simulink model "c00010M_harness"  (R2018a)
settings: Solver=ode3  StartTime=0.0  StopTime=10.0  RelTol=1e-3  EnableMultiTasking=on
undefined symbols (not defined in the file): b, DiscIntNeverNeededParam, J, K, L, PosMinimaW3, R, sigbuilder_block
(part 18 of 43)

== system c00010M_harness/M036/Physical/W ==
  WIn : Inport
  DC_Engine : Subsystem
  Discrete-Time Integrator : DiscreteIntegrator  InitialCondition=5  SampleTime=-1  LimitOutput=on  UpperSaturationLimit=5  LowerSaturationLimit=0  ICPrevOutput=DiscIntNeverNeededParam  ICPrevScaledInput=DiscIntNeverNeededParam
  WPos : Outport
  wires:
  WIn/1 -> DC_Engine/1(input)
  DC_Engine/1(Speed) -> Discrete-Time Integrator/1
  Discrete-Time Integrator/1 -> WPos/1

== system c00010M_harness/M036/Physical/W5 ==
  WIn : Inport
  DC_Engine : Subsystem
  Discrete-Time Integrator : DiscreteIntegrator  InitialCondition=5  SampleTime=-1  LimitOutput=on  UpperSaturationLimit=5  LowerSaturationLimit=0  ICPrevOutput=DiscIntNeverNeededParam  ICPrevScaledInput=DiscIntNeverNeededParam
  WPos : Outport
  wires:
  Discrete-Time Integrator/1 -> WPos/1
  DC_Engine/1(Speed) -> Discrete-Time Integrator/1
  WIn/1 -> DC_Engine/1(input)

== system c00010M_harness/M036/Physical/W6 ==
  WIn : Inport
  DC_Engine : Subsystem
  Discrete-Time Integrator : DiscreteIntegrator  InitialCondition=5  SampleTime=-1  LimitOutput=on  UpperSaturationLimit=5  LowerSaturationLimit=PosMinimaW3  ICPrevOutput=DiscIntNeverNeededParam  ICPrevScaledInput=DiscIntNeverNeededParam
  WPos : Outport
  wires:
  WIn/1 -> DC_Engine/1(input)
  DC_Engine/1(Speed) -> Discrete-Time Integrator/1
  Discrete-Time Integrator/1 -> WPos/1

== system c00010M_harness/M037/Cyber/Pri ==
  D : Inport
  P : Inport  Port=2
  Switch : Switch  Criteria=u2 ~= 0
  User : Outport
  wires:
  Switch/1 -> User/1
  D/1 -> Switch/2, Switch/1
  P/1 -> Switch/3

== system c00010M_harness/M037/Cyber/Pri1 ==
  D : Inport
  P : Inport  Port=2
  P1 : Inport  Port=3
  Switch : Switch  Criteria=u2 ~= 0
  Switch1 : Switch  Criteria=u2 ~= 0
  User : Outport
  wires:
  Switch1/1 -> Switch/3
  D/1 -> Switch/2, Switch/1
  P/1 -> Switch1/2, Switch1/1
  Switch/1 -> User/1
  P1/1 -> Switch1/3

== system c00010M_harness/M037/Cyber/WL ==
  note: Sensors
  WPos : Inport
  User : Inport  Port=2
  OW : Inport  Port=3
  Chart : Stateflow chart  TreatAsAtomicUnit=on
  Constant : Constant  Value=-1
  Data Type Conversion : DataTypeConversion
  Switch : Switch  Criteria=u2 ~= 0  Threshold=1  ZeroCross=off
  WindowLogicOutput : Outport
  wires:
  Data Type Conversion/1 -> Switch/2
  Constant/1 -> Switch/1
  User/1 -> Chart/2(UI)
  WPos/1 -> Chart/1(S)
  Switch/1 -> WindowLogicOutput/1
  OW/1 -> Data Type Conversion/1
  Chart/1(W) -> Switch/3

== system c00010M_harness/M037/Cyber/WL1 ==
  note: Sensors
  WPos : Inport
  User : Inport  Port=2
  OW : Inport  Port=3
  Chart1 : Stateflow chart  TreatAsAtomicUnit=on
  Constant : Constant  Value=-1
  Data Type Conversion : DataTypeConversion
  Switch : Switch  Criteria=u2 ~= 0  Threshold=1  ZeroCross=off
  WindowLogicOutput : Outport
  wires:
  OW/1 -> Data Type Conversion/1
  Switch/1 -> WindowLogicOutput/1
  WPos/1 -> Chart1/1(S)
  User/1 -> Chart1/2(UI)
  Constant/1 -> Switch/1
  Data Type Conversion/1 -> Switch/2
  Chart1/1(W) -> Switch/3

== system c00010M_harness/M037/Cyber/WL2 ==
  note: Sensors
  WPos : Inport
  User : Inport  Port=2
  OW : Inport  Port=3
  L : Inport  Port=4
  Chart1 : Stateflow chart  TreatAsAtomicUnit=on
  Constant : Constant  Value=-1
  Constant1 : Constant  Value=0
  Constant2 : Constant  Value=PosMinimaW3
  Data Type Conversion : DataTypeConversion
  Switch : Switch  Criteria=u2 ~= 0  Threshold=1  ZeroCross=off
  Switch1 : Switch  Criteria=u2 ~= 0
  WindowLogicOutput : Outport
  wires:
  Constant2/1 -> Chart1/3(PosMinW3)
  L/1 -> Switch1/2
  Data Type Conversion/1 -> Switch/2
  Constant/1 -> Switch/1
  Chart1/1(W) -> Switch1/3
  User/1 -> Chart1/2(UI)
  WPos/1 -> Chart1/1(S)
  Switch1/1 -> Switch/3
  Constant1/1 -> Switch1/1
  Switch/1 -> WindowLogicOutput/1
  OW/1 -> Data Type Conversion/1

== system c00010M_harness/M037/Physical/W ==
  WIn : Inport
  DC_Engine : Subsystem
  Discrete-Time Integrator : DiscreteIntegrator  InitialCondition=5  SampleTime=-1  LimitOutput=on  UpperSaturationLimit=5  LowerSaturationLimit=0  ICPrevOutput=DiscIntNeverNeededParam  ICPrevScaledInput=DiscIntNeverNeededParam
  WPos : Outport
  wires:
  WIn/1 -> DC_Engine/1(input)
  DC_Engine/1(Speed) -> Discrete-Time Integrator/1
  Discrete-Time Integrator/1 -> WPos/1

== system c00010M_harness/M037/Physical/W5 ==
  WIn : Inport
  DC_Engine : Subsystem
  Discrete-Time Integrator : DiscreteIntegrator  InitialCondition=5  SampleTime=-1  LimitOutput=on  UpperSaturationLimit=5  LowerSaturationLimit=0  ICPrevOutput=DiscIntNeverNeededParam  ICPrevScaledInput=DiscIntNeverNeededParam
  WPos : Outport
  wires:
  Discrete-Time Integrator/1 -> WPos/1
  DC_Engine/1(Speed) -> Discrete-Time Integrator/1
  WIn/1 -> DC_Engine/1(input)

== system c00010M_harness/M037/Physical/W6 ==
  WIn : Inport
  DC_Engine : Subsystem
  Discrete-Time Integrator : DiscreteIntegrator  InitialCondition=5  SampleTime=-1  LimitOutput=on  UpperSaturationLimit=5  LowerSaturationLimit=PosMinimaW3  ICPrevOutput=DiscIntNeverNeededParam  ICPrevScaledInput=DiscIntNeverNeededParam
  WPos : Outport
  wires:
  WIn/1 -> DC_Engine/1(input)
  DC_Engine/1(Speed) -> Discrete-Time Integrator/1
  Discrete-Time Integrator/1 -> WPos/1

== system c00010M_harness/M039/Cyber/Pri ==
  D : Inport
  P : Inport  Port=2
  Switch : Switch  Criteria=u2 ~= 0
  User : Outport
  wires:
  Switch/1 -> User/1
  D/1 -> Switch/2, Switch/1
  P/1 -> Switch/3

== system c00010M_harness/M039/Cyber/Pri1 ==
  D : Inport
  P : Inport  Port=2
  P1 : Inport  Port=3
  Switch : Switch  Criteria=u2 ~= 0
  Switch1 : Switch  Criteria=u2 ~= 0
  User : Outport
  wires:
  Switch1/1 -> Switch/3
  D/1 -> Switch/2, Switch/1
  P/1 -> Switch1/2, Switch1/1
  Switch/1 -> User/1
  P1/1 -> Switch1/3

== system c00010M_harness/M039/Cyber/WL ==
  note: Sensors
  WPos : Inport
  User : Inport  Port=2
  OW : Inport  Port=3
  Chart : Stateflow chart  TreatAsAtomicUnit=on
  Constant : Constant  Value=-1
  Data Type Conversion : DataTypeConversion
  Switch : Switch  Criteria=u2 ~= 0  Threshold=1  ZeroCross=off
  WindowLogicOutput : Outport
  wires:
  Data Type Conversion/1 -> Switch/2
  Constant/1 -> Switch/1
  User/1 -> Chart/2(UI)
  WPos/1 -> Chart/1(S)
  Switch/1 -> WindowLogicOutput/1
  OW/1 -> Data Type Conversion/1
  Chart/1(W) -> Switch/3

== system c00010M_harness/M039/Cyber/WL1 ==
  note: Sensors
  WPos : Inport
  User : Inport  Port=2
  OW : Inport  Port=3
  Chart1 : Stateflow chart  TreatAsAtomicUnit=on
  Constant : Constant  Value=-1
  Data Type Conversion : DataTypeConversion
  Switch : Switch  Criteria=u2 ~= 0  Threshold=1  ZeroCross=off
  WindowLogicOutput : Outport
  wires:
  OW/1 -> Data Type Conversion/1
  Switch/1 -> WindowLogicOutput/1
  WPos/1 -> Chart1/1(S)
  User/1 -> Chart1/2(UI)
  Constant/1 -> Switch/1
  Data Type Conversion/1 -> Switch/2
  Chart1/1(W) -> Switch/3

== system c00010M_harness/M039/Cyber/WL2 ==
  note: Sensors
  WPos : Inport
  User : Inport  Port=2
  OW : Inport  Port=3
  L : Inport  Port=4
  Chart1 : Stateflow chart  TreatAsAtomicUnit=on
  Constant : Constant  Value=-1
  Constant1 : Constant  Value=0
  Constant2 : Constant  Value=PosMinimaW3
  Data Type Conversion : DataTypeConversion
  Switch : Switch  Criteria=u2 ~= 0  Threshold=1  ZeroCross=off
  Switch1 : Switch  Criteria=u2 ~= 0
  WindowLogicOutput : Outport
  wires:
  Constant2/1 -> Chart1/3(PosMinW3)
  L/1 -> Switch1/2
  Data Type Conversion/1 -> Switch/2
  Constant/1 -> Switch/1
  Chart1/1(W) -> Switch1/3
  User/1 -> Chart1/2(UI)
  WPos/1 -> Chart1/1(S)
  Switch1/1 -> Switch/3
  Constant1/1 -> Switch1/1
  Switch/1 -> WindowLogicOutput/1
  OW/1 -> Data Type Conversion/1

== system c00010M_harness/M039/Physical/W ==
  WIn : Inport
  DC_Engine : Subsystem
  Discrete-Time Integrator : DiscreteIntegrator  InitialCondition=5  SampleTime=-1  LimitOutput=on  UpperSaturationLimit=5  LowerSaturationLimit=0  ICPrevOutput=DiscIntNeverNeededParam  ICPrevScaledInput=DiscIntNeverNeededParam
  WPos : Outport
  wires:
  WIn/1 -> DC_Engine/1(input)
  DC_Engine/1(Speed) -> Discrete-Time Integrator/1
  Discrete-Time Integrator/1 -> WPos/1

== system c00010M_harness/M039/Physical/W5 ==
  WIn : Inport
  DC_Engine : Subsystem
  Discrete-Time Integrator : DiscreteIntegrator  InitialCondition=5  SampleTime=-1  LimitOutput=on  UpperSaturationLimit=5  LowerSaturationLimit=0  ICPrevOutput=DiscIntNeverNeededParam  ICPrevScaledInput=DiscIntNeverNeededParam
  WPos : Outport
  wires:
  Discrete-Time Integrator/1 -> WPos/1
  DC_Engine/1(Speed) -> Discrete-Time Integrator/1
  WIn/1 -> DC_Engine/1(input)

== system c00010M_harness/M039/Physical/W6 ==
  WIn : Inport
  DC_Engine : Subsystem
  Discrete-Time Integrator : DiscreteIntegrator  InitialCondition=5  SampleTime=-1  LimitOutput=on  UpperSaturationLimit=5  LowerSaturationLimit=PosMinimaW3  ICPrevOutput=DiscIntNeverNeededParam  ICPrevScaledInput=DiscIntNeverNeededParam
  WPos : Outport
  wires:
  WIn/1 -> DC_Engine/1(input)
  DC_Engine/1(Speed) -> Discrete-Time Integrator/1
  Discrete-Time Integrator/1 -> WPos/1

== system c00010M_harness/M040/Cyber/Pri ==
  D : Inport
  P : Inport  Port=2
  Switch : Switch  Criteria=u2 ~= 0
  User : Outport
  wires:
  Switch/1 -> User/1
  D/1 -> Switch/2, Switch/1
  P/1 -> Switch/3

== system c00010M_harness/M040/Cyber/Pri1 ==
  D : Inport
  P : Inport  Port=2
  P1 : Inport  Port=3
  Switch : Switch  Criteria=u2 ~= 0
  Switch1 : Switch  Criteria=u2 ~= 0
  User : Outport
  wires:
  Switch1/1 -> Switch/3
  D/1 -> Switch/2, Switch/1
  P/1 -> Switch1/2, Switch1/1
  Switch/1 -> User/1
  P1/1 -> Switch1/3

== system c00010M_harness/M040/Cyber/WL ==
  note: Sensors
  WPos : Inport
  User : Inport  Port=2
  OW : Inport  Port=3
  Chart : Stateflow chart  TreatAsAtomicUnit=on
  Constant : Constant  Value=-1
  Data Type Conversion : DataTypeConversion
  Switch : Switch  Criteria=u2 ~= 0  Threshold=1  ZeroCross=off
  WindowLogicOutput : Outport
  wires:
  Data Type Conversion/1 -> Switch/2
  Constant/1 -> Switch/1
  User/1 -> Chart/2(UI)
  WPos/1 -> Chart/1(S)
  Switch/1 -> WindowLogicOutput/1
  OW/1 -> Data Type Conversion/1
  Chart/1(W) -> Switch/3

== system c00010M_harness/M040/Cyber/WL1 ==
  note: Sensors
  WPos : Inport
  User : Inport  Port=2
  OW : Inport  Port=3
  Chart1 : Stateflow chart  TreatAsAtomicUnit=on
  Constant : Constant  Value=-1
  Data Type Conversion : DataTypeConversion
  Switch : Switch  Criteria=u2 ~= 0  Threshold=1  ZeroCross=off
  WindowLogicOutput : Outport
  wires:
  OW/1 -> Data Type Conversion/1
  Switch/1 -> WindowLogicOutput/1
  WPos/1 -> Chart1/1(S)
  User/1 -> Chart1/2(UI)
  Constant/1 -> Switch/1
  Data Type Conversion/1 -> Switch/2
  Chart1/1(W) -> Switch/3

== system c00010M_harness/M040/Cyber/WL2 ==
  note: Sensors
  WPos : Inport
  User : Inport  Port=2
  OW : Inport  Port=3
  L : Inport  Port=4
  Chart1 : Stateflow chart  TreatAsAtomicUnit=on
  Constant : Constant  Value=-1
  Constant1 : Constant  Value=0
  Constant2 : Constant  Value=PosMinimaW3
  Data Type Conversion : DataTypeConversion
  Switch : Switch  Criteria=u2 ~= 0  Threshold=1  ZeroCross=off
  Switch1 : Switch  Criteria=u2 ~= 0
  WindowLogicOutput : Outport
  wires:
  Constant2/1 -> Chart1/3(PosMinW3)
  L/1 -> Switch1/2
  Data Type Conversion/1 -> Switch/2
  Constant/1 -> Switch/1
  Chart1/1(W) -> Switch1/3
  User/1 -> Chart1/2(UI)
  WPos/1 -> Chart1/1(S)
  Switch1/1 -> Switch/3
  Constant1/1 -> Switch1/1
  Switch/1 -> WindowLogicOutput/1
  OW/1 -> Data Type Conversion/1

== system c00010M_harness/M040/Physical/W ==
  WIn : Inport
  DC_Engine : Subsystem
  Discrete-Time Integrator : DiscreteIntegrator  InitialCondition=5  SampleTime=-1  LimitOutput=on  UpperSaturationLimit=5  LowerSaturationLimit=0  ICPrevOutput=DiscIntNeverNeededParam  ICPrevScaledInput=DiscIntNeverNeededParam
  WPos : Outport
  wires:
  WIn/1 -> DC_Engine/1(input)
  DC_Engine/1(Speed) -> Discrete-Time Integrator/1
  Discrete-Time Integrator/1 -> WPos/1

== system c00010M_harness/M040/Physical/W5 ==
  WIn : Inport
  DC_Engine : Subsystem
  Discrete-Time Integrator : DiscreteIntegrator  InitialCondition=5  SampleTime=-1  LimitOutput=on  UpperSaturationLimit=5  LowerSaturationLimit=0  ICPrevOutput=DiscIntNeverNeededParam  ICPrevScaledInput=DiscIntNeverNeededParam
  WPos : Outport
  wires:
  Discrete-Time Integrator/1 -> WPos/1
  DC_Engine/1(Speed) -> Discrete-Time Integrator/1
  WIn/1 -> DC_Engine/1(input)

== system c00010M_harness/M040/Physical/W6 ==
  WIn : Inport
  DC_Engine : Subsystem
  Discrete-Time Integrator : DiscreteIntegrator  InitialCondition=5  SampleTime=-1  LimitOutput=on  UpperSaturationLimit=5  LowerSaturationLimit=PosMinimaW3  ICPrevOutput=DiscIntNeverNeededParam  ICPrevScaledInput=DiscIntNeverNeededParam
  WPos : Outport
  wires:
  WIn/1 -> DC_Engine/1(input)
  DC_Engine/1(Speed) -> Discrete-Time Integrator/1
  Discrete-Time Integrator/1 -> WPos/1

== system c00010M_harness/M041/Cyber/Pri ==
  D : Inport
  P : Inport  Port=2
  Switch : Switch  Criteria=u2 ~= 0
  User : Outport
  wires:
  Switch/1 -> User/1
  D/1 -> Switch/2, Switch/1
  P/1 -> Switch/3

== system c00010M_harness/M041/Cyber/Pri1 ==
  D : Inport
  P : Inport  Port=2
  P1 : Inport  Port=3
  Switch : Switch  Criteria=u2 ~= 0
  Switch1 : Switch  Criteria=u2 ~= 0
  User : Outport
  wires:
  Switch1/1 -> Switch/3
  D/1 -> Switch/2, Switch/1
  P/1 -> Switch1/2, Switch1/1
  Switch/1 -> User/1
  P1/1 -> Switch1/3

== system c00010M_harness/M041/Cyber/WL ==
  note: Sensors
  WPos : Inport
  User : Inport  Port=2
  OW : Inport  Port=3
  Chart : Stateflow chart  TreatAsAtomicUnit=on
  Constant : Constant  Value=-1
  Data Type Conversion : DataTypeConversion
  Switch : Switch  Criteria=u2 ~= 0  Threshold=1  ZeroCross=off
  WindowLogicOutput : Outport
  wires:
  Data Type Conversion/1 -> Switch/2
  Constant/1 -> Switch/1
  User/1 -> Chart/2(UI)
  WPos/1 -> Chart/1(S)
  Switch/1 -> WindowLogicOutput/1
  OW/1 -> Data Type Conversion/1
  Chart/1(W) -> Switch/3

== system c00010M_harness/M041/Cyber/WL1 ==
  note: Sensors
  WPos : Inport
  User : Inport  Port=2
  OW : Inport  Port=3
  Chart1 : Stateflow chart  TreatAsAtomicUnit=on
  Constant : Constant  Value=-1
  Data Type Conversion : DataTypeConversion
  Switch : Switch  Criteria=u2 ~= 0  Threshold=1  ZeroCross=off
  WindowLogicOutput : Outport
  wires:
  OW/1 -> Data Type Conversion/1
  Switch/1 -> WindowLogicOutput/1
  WPos/1 -> Chart1/1(S)
  User/1 -> Chart1/2(UI)
  Constant/1 -> Switch/1
  Data Type Conversion/1 -> Switch/2
  Chart1/1(W) -> Switch/3

== system c00010M_harness/M041/Cyber/WL2 ==
  note: Sensors
  WPos : Inport
  User : Inport  Port=2
  OW : Inport  Port=3
  L : Inport  Port=4
  Chart1 : Stateflow chart  TreatAsAtomicUnit=on
  Constant : Constant  Value=-1
  Constant1 : Constant  Value=0
  Constant2 : Constant  Value=PosMinimaW3
  Data Type Conversion : DataTypeConversion
  Switch : Switch  Criteria=u2 ~= 0  Threshold=1  ZeroCross=off
  Switch1 : Switch  Criteria=u2 ~= 0
  WindowLogicOutput : Outport
  wires:
  Constant2/1 -> Chart1/3(PosMinW3)
  L/1 -> Switch1/2
  Data Type Conversion/1 -> Switch/2
  Constant/1 -> Switch/1
  Chart1/1(W) -> Switch1/3
  User/1 -> Chart1/2(UI)
  WPos/1 -> Chart1/1(S)
  Switch1/1 -> Switch/3
  Constant1/1 -> Switch1/1
  Switch/1 -> WindowLogicOutput/1
  OW/1 -> Data Type Conversion/1

== system c00010M_harness/M041/Physical/W ==
  WIn : Inport
  DC_Engine : Subsystem
  Discrete-Time Integrator : DiscreteIntegrator  InitialCondition=5  SampleTime=-1  LimitOutput=on  UpperSaturationLimit=5  LowerSaturationLimit=0  ICPrevOutput=DiscIntNeverNeededParam  ICPrevScaledInput=DiscIntNeverNeededParam
  WPos : Outport
  wires:
  WIn/1 -> DC_Engine/1(input)
  DC_Engine/1(Speed) -> Discrete-Time Integrator/1
  Discrete-Time Integrator/1 -> WPos/1

== system c00010M_harness/M041/Physical/W5 ==
  WIn : Inport
  DC_Engine : Subsystem
  Discrete-Time Integrator : DiscreteIntegrator  InitialCondition=5  SampleTime=-1  LimitOutput=on  UpperSaturationLimit=5  LowerSaturationLimit=0  ICPrevOutput=DiscIntNeverNeededParam  ICPrevScaledInput=DiscIntNeverNeededParam
  WPos : Outport
  wires:
  Discrete-Time Integrator/1 -> WPos/1
  DC_Engine/1(Speed) -> Discrete-Time Integrator/1
  WIn/1 -> DC_Engine/1(input)

== system c00010M_harness/M041/Physical/W6 ==
  WIn : Inport
  DC_Engine : Subsystem
  Discrete-Time Integrator : DiscreteIntegrator  InitialCondition=5  SampleTime=-1  LimitOutput=on  UpperSaturationLimit=5  LowerSaturationLimit=PosMinimaW3  ICPrevOutput=DiscIntNeverNeededParam  ICPrevScaledInput=DiscIntNeverNeededParam
  WPos : Outport
  wires:
  WIn/1 -> DC_Engine/1(input)
  DC_Engine/1(Speed) -> Discrete-Time Integrator/1
  Discrete-Time Integrator/1 -> WPos/1

== system c00010M_harness/M043/Cyber/Pri ==
  D : Inport
  P : Inport  Port=2
  Switch : Switch  Criteria=u2 ~= 0
  User : Outport
  wires:
  Switch/1 -> User/1
  D/1 -> Switch/2, Switch/1
  P/1 -> Switch/3

== system c00010M_harness/M043/Cyber/Pri1 ==
  D : Inport
  P : Inport  Port=2
  P1 : Inport  Port=3
  Switch : Switch  Criteria=u2 ~= 0
  Switch1 : Switch  Criteria=u2 ~= 0
  User : Outport
  wires:
  Switch1/1 -> Switch/3
  D/1 -> Switch/2, Switch/1
  P/1 -> Switch1/2, Switch1/1
  Switch/1 -> User/1
  P1/1 -> Switch1/3

== system c00010M_harness/M043/Cyber/WL ==
  note: Sensors
  WPos : Inport
  User : Inport  Port=2
  OW : Inport  Port=3
  Chart : Stateflow chart  TreatAsAtomicUnit=on
  Constant : Constant  Value=-1
  Data Type Conversion : DataTypeConversion
  Switch : Switch  Criteria=u2 ~= 0  Threshold=1  ZeroCross=off
  WindowLogicOutput : Outport
  wires:
  Data Type Conversion/1 -> Switch/2
  Constant/1 -> Switch/1
  User/1 -> Chart/2(UI)
  WPos/1 -> Chart/1(S)
  Switch/1 -> WindowLogicOutput/1
  OW/1 -> Data Type Conversion/1
  Chart/1(W) -> Switch/3

== system c00010M_harness/M043/Cyber/WL1 ==
  note: Sensors
  WPos : Inport
  User : Inport  Port=2
  OW : Inport  Port=3
  Chart1 : Stateflow chart  TreatAsAtomicUnit=on
  Constant : Constant  Value=-1
  Data Type Conversion : DataTypeConversion
  Switch : Switch  Criteria=u2 ~= 0  Threshold=1  ZeroCross=off
  WindowLogicOutput : Outport
  wires:
  OW/1 -> Data Type Conversion/1
  Switch/1 -> WindowLogicOutput/1
  WPos/1 -> Chart1/1(S)
  User/1 -> Chart1/2(UI)
  Constant/1 -> Switch/1
  Data Type Conversion/1 -> Switch/2
  Chart1/1(W) -> Switch/3

== system c00010M_harness/M043/Cyber/WL2 ==
  note: Sensors
  WPos : Inport
  User : Inport  Port=2
  OW : Inport  Port=3
  L : Inport  Port=4
  Chart1 : Stateflow chart  TreatAsAtomicUnit=on
  Constant : Constant  Value=-1
  Constant1 : Constant  Value=0
  Constant2 : Constant  Value=PosMinimaW3
  Data Type Conversion : DataTypeConversion
  Switch : Switch  Criteria=u2 ~= 0  Threshold=1  ZeroCross=off
  Switch1 : Switch  Criteria=u2 ~= 0
  WindowLogicOutput : Outport
  wires:
  Constant2/1 -> Chart1/3(PosMinW3)
  L/1 -> Switch1/2
  Data Type Conversion/1 -> Switch/2
  Constant/1 -> Switch/1
  Chart1/1(W) -> Switch1/3
  User/1 -> Chart1/2(UI)
  WPos/1 -> Chart1/1(S)
  Switch1/1 -> Switch/3
  Constant1/1 -> Switch1/1
  Switch/1 -> WindowLogicOutput/1
  OW/1 -> Data Type Conversion/1

== system c00010M_harness/M043/Physical/W ==
  WIn : Inport
  DC_Engine : Subsystem
  Discrete-Time Integrator : DiscreteIntegrator  InitialCondition=5  SampleTime=-1  LimitOutput=on  UpperSaturationLimit=5  LowerSaturationLimit=0  ICPrevOutput=DiscIntNeverNeededParam  ICPrevScaledInput=DiscIntNeverNeededParam
  WPos : Outport
  wires:
  WIn/1 -> DC_Engine/1(input)
  DC_Engine/1(Speed) -> Discrete-Time Integrator/1
  Discrete-Time Integrator/1 -> WPos/1

== system c00010M_harness/M043/Physical/W5 ==
  WIn : Inport
  DC_Engine : Subsystem
  Discrete-Time Integrator : DiscreteIntegrator  InitialCondition=5  SampleTime=-1  LimitOutput=on  UpperSaturationLimit=5  LowerSaturationLimit=0  ICPrevOutput=DiscIntNeverNeededParam  ICPrevScaledInput=DiscIntNeverNeededParam
  WPos : Outport
  wires:
  Discrete-Time Integrator/1 -> WPos/1
  DC_Engine/1(Speed) -> Discrete-Time Integrator/1
  WIn/1 -> DC_Engine/1(input)

== system c00010M_harness/M043/Physical/W6 ==
  WIn : Inport
  DC_Engine : Subsystem
  Discrete-Time Integrator : DiscreteIntegrator  InitialCondition=5  SampleTime=-1  LimitOutput=on  UpperSaturationLimit=5  LowerSaturationLimit=PosMinimaW3  ICPrevOutput=DiscIntNeverNeededParam  ICPrevScaledInput=DiscIntNeverNeededParam
  WPos : Outport
  wires:
  WIn/1 -> DC_Engine/1(input)
  DC_Engine/1(Speed) -> Discrete-Time Integrator/1
  Discrete-Time Integrator/1 -> WPos/1

== system c00010M_harness/M044/Cyber/Pri ==
  D : Inport
  P : Inport  Port=2
  Switch : Switch  Criteria=u2 ~= 0
  User : Outport
  wires:
  Switch/1 -> User/1
  D/1 -> Switch/2, Switch/1
  P/1 -> Switch/3

== system c00010M_harness/M044/Cyber/Pri1 ==
  D : Inport
  P : Inport  Port=2
  P1 : Inport  Port=3
  Switch : Switch  Criteria=u2 ~= 0
  Switch1 : Switch  Criteria=u2 ~= 0
  User : Outport
  wires:
  Switch1/1 -> Switch/3
  D/1 -> Switch/2, Switch/1
  P/1 -> Switch1/2, Switch1/1
  Switch/1 -> User/1
  P1/1 -> Switch1/3

== system c00010M_harness/M044/Cyber/WL ==
  note: Sensors
  WPos : Inport
  User : Inport  Port=2
  OW : Inport  Port=3
  Chart : Stateflow chart  TreatAsAtomicUnit=on
  Constant : Constant  Value=-1
  Data Type Conversion : DataTypeConversion
  Switch : Switch  Criteria=u2 ~= 0  Threshold=1  ZeroCross=off
  WindowLogicOutput : Outport
  wires:
  Data Type Conversion/1 -> Switch/2
  Constant/1 -> Switch/1
  User/1 -> Chart/2(UI)
  WPos/1 -> Chart/1(S)
  Switch/1 -> WindowLogicOutput/1
  OW/1 -> Data Type Conversion/1
  Chart/1(W) -> Switch/3

== system c00010M_harness/M044/Cyber/WL1 ==
  note: Sensors
  WPos : Inport
  User : Inport  Port=2
  OW : Inport  Port=3
  Chart1 : Stateflow chart  TreatAsAtomicUnit=on
  Constant : Constant  Value=-1
  Data Type Conversion : DataTypeConversion
  Switch : Switch  Criteria=u2 ~= 0  Threshold=1  ZeroCross=off
  WindowLogicOutput : Outport
  wires:
  OW/1 -> Data Type Conversion/1
  Switch/1 -> WindowLogicOutput/1
  WPos/1 -> Chart1/1(S)
  User/1 -> Chart1/2(UI)
  Constant/1 -> Switch/1
  Data Type Conversion/1 -> Switch/2
  Chart1/1(W) -> Switch/3

== system c00010M_harness/M044/Cyber/WL2 ==
  note: Sensors
  WPos : Inport
  User : Inport  Port=2
  OW : Inport  Port=3
  L : Inport  Port=4
  Chart1 : Stateflow chart  TreatAsAtomicUnit=on
  Constant : Constant  Value=-1
  Constant1 : Constant  Value=0
  Constant2 : Constant  Value=PosMinimaW3
  Data Type Conversion : DataTypeConversion
  Switch : Switch  Criteria=u2 ~= 0  Threshold=1  ZeroCross=off
  Switch1 : Switch  Criteria=u2 ~= 0
  WindowLogicOutput : Outport
  wires:
  Constant2/1 -> Chart1/3(PosMinW3)
  L/1 -> Switch1/2
  Data Type Conversion/1 -> Switch/2
  Constant/1 -> Switch/1
  Chart1/1(W) -> Switch1/3
  User/1 -> Chart1/2(UI)
  WPos/1 -> Chart1/1(S)
  Switch1/1 -> Switch/3
  Constant1/1 -> Switch1/1
  Switch/1 -> WindowLogicOutput/1
  OW/1 -> Data Type Conversion/1

== system c00010M_harness/M044/Physical/W ==
  WIn : Inport
  DC_Engine : Subsystem
  Discrete-Time Integrator : DiscreteIntegrator  InitialCondition=5  SampleTime=-1  LimitOutput=on  UpperSaturationLimit=5  LowerSaturationLimit=0  ICPrevOutput=DiscIntNeverNeededParam  ICPrevScaledInput=DiscIntNeverNeededParam
  WPos : Outport
  wires:
  WIn/1 -> DC_Engine/1(input)
  DC_Engine/1(Speed) -> Discrete-Time Integrator/1
  Discrete-Time Integrator/1 -> WPos/1

== system c00010M_harness/M044/Physical/W5 ==
  WIn : Inport
  DC_Engine : Subsystem
  Discrete-Time Integrator : DiscreteIntegrator  InitialCondition=5  SampleTime=-1  LimitOutput=on  UpperSaturationLimit=5  LowerSaturationLimit=0  ICPrevOutput=DiscIntNeverNeededParam  ICPrevScaledInput=DiscIntNeverNeededParam
  WPos : Outport
  wires:
  Discrete-Time Integrator/1 -> WPos/1
  DC_Engine/1(Speed) -> Discrete-Time Integrator/1
  WIn/1 -> DC_Engine/1(input)

== system c00010M_harness/M044/Physical/W6 ==
  WIn : Inport
  DC_Engine : Subsystem
  Discrete-Time Integrator : DiscreteIntegrator  InitialCondition=5  SampleTime=-1  LimitOutput=on  UpperSaturationLimit=5  LowerSaturationLimit=PosMinimaW3  ICPrevOutput=DiscIntNeverNeededParam  ICPrevScaledInput=DiscIntNeverNeededParam
  WPos : Outport
  wires:
  WIn/1 -> DC_Engine/1(input)
  DC_Engine/1(Speed) -> Discrete-Time Integrator/1
  Discrete-Time Integrator/1 -> WPos/1

== system c00010M_harness/M045/Cyber/Pri ==
  D : Inport
  P : Inport  Port=2
  Switch : Switch  Criteria=u2 ~= 0
  User : Outport
  wires:
  Switch/1 -> User/1
  D/1 -> Switch/2, Switch/1
  P/1 -> Switch/3

== system c00010M_harness/M045/Cyber/Pri1 ==
  D : Inport
  P : Inport  Port=2
  P1 : Inport  Port=3
  Switch : Switch  Criteria=u2 ~= 0
  Switch1 : Switch  Criteria=u2 ~= 0
  User : Outport
  wires:
  Switch1/1 -> Switch/3
  D/1 -> Switch/2, Switch/1
  P/1 -> Switch1/2, Switch1/1
  Switch/1 -> User/1
  P1/1 -> Switch1/3

== system c00010M_harness/M045/Cyber/WL ==
  note: Sensors
  WPos : Inport
  User : Inport  Port=2
  OW : Inport  Port=3
  Chart : Stateflow chart  TreatAsAtomicUnit=on
  Constant : Constant  Value=-1
  Data Type Conversion : DataTypeConversion
  Switch : Switch  Criteria=u2 ~= 0  Threshold=1  ZeroCross=off
  WindowLogicOutput : Outport
  wires:
  Data Type Conversion/1 -> Switch/2
  Constant/1 -> Switch/1
  User/1 -> Chart/2(UI)
  WPos/1 -> Chart/1(S)
  Switch/1 -> WindowLogicOutput/1
  OW/1 -> Data Type Conversion/1
  Chart/1(W) -> Switch/3

== system c00010M_harness/M045/Cyber/WL1 ==
  note: Sensors
  WPos : Inport
  User : Inport  Port=2
  OW : Inport  Port=3
  Chart1 : Stateflow chart  TreatAsAtomicUnit=on
  Constant : Constant  Value=-1
  Data Type Conversion : DataTypeConversion
  Switch : Switch  Criteria=u2 ~= 0  Threshold=1  ZeroCross=off
  WindowLogicOutput : Outport
  wires:
  OW/1 -> Data Type Conversion/1
  Switch/1 -> WindowLogicOutput/1
  WPos/1 -> Chart1/1(S)
  User/1 -> Chart1/2(UI)
  Constant/1 -> Switch/1
  Data Type Conversion/1 -> Switch/2
  Chart1/1(W) -> Switch/3

== system c00010M_harness/M045/Cyber/WL2 ==
  note: Sensors
  WPos : Inport
  User : Inport  Port=2
  OW : Inport  Port=3
  L : Inport  Port=4
  Chart1 : Stateflow chart  TreatAsAtomicUnit=on
  Constant : Constant  Value=-1
  Constant1 : Constant  Value=0
  Constant2 : Constant  Value=PosMinimaW3
  Data Type Conversion : DataTypeConversion
  Switch : Switch  Criteria=u2 ~= 0  Threshold=1  ZeroCross=off
  Switch1 : Switch  Criteria=u2 ~= 0
  WindowLogicOutput : Outport
  wires:
  Constant2/1 -> Chart1/3(PosMinW3)
  L/1 -> Switch1/2
  Data Type Conversion/1 -> Switch/2
  Constant/1 -> Switch/1
  Chart1/1(W) -> Switch1/3
  User/1 -> Chart1/2(UI)
  WPos/1 -> Chart1/1(S)
  Switch1/1 -> Switch/3
  Constant1/1 -> Switch1/1
  Switch/1 -> WindowLogicOutput/1
  OW/1 -> Data Type Conversion/1

== system c00010M_harness/M045/Physical/W ==
  WIn : Inport
  DC_Engine : Subsystem
  Discrete-Time Integrator : DiscreteIntegrator  InitialCondition=5  SampleTime=-1  LimitOutput=on  UpperSaturationLimit=5  LowerSaturationLimit=0  ICPrevOutput=DiscIntNeverNeededParam  ICPrevScaledInput=DiscIntNeverNeededParam
  WPos : Outport
  wires:
  WIn/1 -> DC_Engine/1(input)
  DC_Engine/1(Speed) -> Discrete-Time Integrator/1
  Discrete-Time Integrator/1 -> WPos/1

== system c00010M_harness/M045/Physical/W5 ==
  WIn : Inport
  DC_Engine : Subsystem
  Discrete-Time Integrator : DiscreteIntegrator  InitialCondition=5  SampleTime=-1  LimitOutput=on  UpperSaturationLimit=5  LowerSaturationLimit=0  ICPrevOutput=DiscIntNeverNeededParam  ICPrevScaledInput=DiscIntNeverNeededParam
  WPos : Outport
  wires:
  Discrete-Time Integrator/1 -> WPos/1
  DC_Engine/1(Speed) -> Discrete-Time Integrator/1
  WIn/1 -> DC_Engine/1(input)

== system c00010M_harness/M045/Physical/W6 ==
  WIn : Inport
  DC_Engine : Subsystem
  Discrete-Time Integrator : DiscreteIntegrator  InitialCondition=5  SampleTime=-1  LimitOutput=on  UpperSaturationLimit=5  LowerSaturationLimit=PosMinimaW3  ICPrevOutput=DiscIntNeverNeededParam  ICPrevScaledInput=DiscIntNeverNeededParam
  WPos : Outport
  wires:
  WIn/1 -> DC_Engine/1(input)
  DC_Engine/1(Speed) -> Discrete-Time Integrator/1
  Discrete-Time Integrator/1 -> WPos/1

== system c00010M_harness/M047/Cyber/Pri ==
  D : Inport
  P : Inport  Port=2
  Switch : Switch  Criteria=u2 ~= 0
  User : Outport
  wires:
  Switch/1 -> User/1
  D/1 -> Switch/2, Switch/1
  P/1 -> Switch/3

== system c00010M_harness/M047/Cyber/Pri1 ==
  D : Inport
  P : Inport  Port=2
  P1 : Inport  Port=3
  Switch : Switch  Criteria=u2 ~= 0
  Switch1 : Switch  Criteria=u2 ~= 0
  User : Outport
  wires:
  Switch1/1 -> Switch/3
  D/1 -> Switch/2, Switch/1
  P/1 -> Switch1/2, Switch1/1
  Switch/1 -> User/1
  P1/1 -> Switch1/3

== system c00010M_harness/M047/Cyber/WL ==
  note: Sensors
  WPos : Inport
  User : Inport  Port=2
  OW : Inport  Port=3
  Chart : Stateflow chart  TreatAsAtomicUnit=on
  Constant : Constant  Value=-1
  Data Type Conversion : DataTypeConversion
  Switch : Switch  Criteria=u2 ~= 0  Threshold=1  ZeroCross=off
  WindowLogicOutput : Outport
  wires:
  Data Type Conversion/1 -> Switch/2
  Constant/1 -> Switch/1
  User/1 -> Chart/2(UI)
  WPos/1 -> Chart/1(S)
  Switch/1 -> WindowLogicOutput/1
  OW/1 -> Data Type Conversion/1
  Chart/1(W) -> Switch/3

== system c00010M_harness/M047/Cyber/WL1 ==
  note: Sensors
  WPos : Inport
  User : Inport  Port=2
  OW : Inport  Port=3
  Chart1 : Stateflow chart  TreatAsAtomicUnit=on
  Constant : Constant  Value=-1
  Data Type Conversion : DataTypeConversion
  Switch : Switch  Criteria=u2 ~= 0  Threshold=1  ZeroCross=off
  WindowLogicOutput : Outport
  wires:
  OW/1 -> Data Type Conversion/1
  Switch/1 -> WindowLogicOutput/1
  WPos/1 -> Chart1/1(S)
  User/1 -> Chart1/2(UI)
  Constant/1 -> Switch/1
  Data Type Conversion/1 -> Switch/2
  Chart1/1(W) -> Switch/3

== system c00010M_harness/M047/Cyber/WL2 ==
  note: Sensors
  WPos : Inport
  User : Inport  Port=2
  OW : Inport  Port=3
  L : Inport  Port=4
  Chart1 : Stateflow chart  TreatAsAtomicUnit=on
  Constant : Constant  Value=-1
  Constant1 : Constant  Value=0
  Constant2 : Constant  Value=PosMinimaW3
  Data Type Conversion : DataTypeConversion
  Switch : Switch  Criteria=u2 ~= 0  Threshold=1  ZeroCross=off
  Switch1 : Switch  Criteria=u2 ~= 0
  WindowLogicOutput : Outport
  wires:
  Constant2/1 -> Chart1/3(PosMinW3)
  L/1 -> Switch1/2
  Data Type Conversion/1 -> Switch/2
  Constant/1 -> Switch/1
  Chart1/1(W) -> Switch1/3
  User/1 -> Chart1/2(UI)
  WPos/1 -> Chart1/1(S)
  Switch1/1 -> Switch/3
  Constant1/1 -> Switch1/1
  Switch/1 -> WindowLogicOutput/1
  OW/1 -> Data Type Conversion/1

== system c00010M_harness/M047/Physical/W ==
  WIn : Inport
  DC_Engine : Subsystem
  Discrete-Time Integrator : DiscreteIntegrator  InitialCondition=5  SampleTime=-1  LimitOutput=on  UpperSaturationLimit=5  LowerSaturationLimit=0  ICPrevOutput=DiscIntNeverNeededParam  ICPrevScaledInput=DiscIntNeverNeededParam
  WPos : Outport
  wires:
  WIn/1 -> DC_Engine/1(input)
  DC_Engine/1(Speed) -> Discrete-Time Integrator/1
  Discrete-Time Integrator/1 -> WPos/1

== system c00010M_harness/M047/Physical/W5 ==
  WIn : Inport
  DC_Engine : Subsystem
  Discrete-Time Integrator : DiscreteIntegrator  InitialCondition=5  SampleTime=-1  LimitOutput=on  UpperSaturationLimit=5  LowerSaturationLimit=0  ICPrevOutput=DiscIntNeverNeededParam  ICPrevScaledInput=DiscIntNeverNeededParam
  WPos : Outport
  wires:
  Discrete-Time Integrator/1 -> WPos/1
  DC_Engine/1(Speed) -> Discrete-Time Integrator/1
  WIn/1 -> DC_Engine/1(input)

== system c00010M_harness/M047/Physical/W6 ==
  WIn : Inport
  DC_Engine : Subsystem
  Discrete-Time Integrator : DiscreteIntegrator  InitialCondition=5  SampleTime=-1  LimitOutput=on  UpperSaturationLimit=5  LowerSaturationLimit=PosMinimaW3  ICPrevOutput=DiscIntNeverNeededParam  ICPrevScaledInput=DiscIntNeverNeededParam
  WPos : Outport
  wires:
  WIn/1 -> DC_Engine/1(input)
  DC_Engine/1(Speed) -> Discrete-Time Integrator/1
  Discrete-Time Integrator/1 -> WPos/1

== system c00010M_harness/M048/Cyber/Pri ==
  D : Inport
  P : Inport  Port=2
  Switch : Switch  Criteria=u2 ~= 0
  User : Outport
  wires:
  Switch/1 -> User/1
  D/1 -> Switch/2, Switch/1
  P/1 -> Switch/3

== system c00010M_harness/M048/Cyber/Pri1 ==
  D : Inport
  P : Inport  Port=2
  P1 : Inport  Port=3
  Switch : Switch  Criteria=u2 ~= 0
  Switch1 : Switch  Criteria=u2 ~= 0
  User : Outport
  wires:
  Switch1/1 -> Switch/3
  D/1 -> Switch/2, Switch/1
  P/1 -> Switch1/2, Switch1/1
  Switch/1 -> User/1
  P1/1 -> Switch1/3

== system c00010M_harness/M048/Cyber/WL ==
  note: Sensors
  WPos : Inport
  User : Inport  Port=2
  OW : Inport  Port=3
  Chart : Stateflow chart  TreatAsAtomicUnit=on
  Constant : Constant  Value=-1
  Data Type Conversion : DataTypeConversion
  Switch : Switch  Criteria=u2 ~= 0  Threshold=1  ZeroCross=off
  WindowLogicOutput : Outport
  wires:
  Data Type Conversion/1 -> Switch/2
  Constant/1 -> Switch/1
  User/1 -> Chart/2(UI)
  WPos/1 -> Chart/1(S)
  Switch/1 -> WindowLogicOutput/1
  OW/1 -> Data Type Conversion/1
  Chart/1(W) -> Switch/3

== system c00010M_harness/M048/Cyber/WL1 ==
  note: Sensors
  WPos : Inport
  User : Inport  Port=2
  OW : Inport  Port=3
  Chart1 : Stateflow chart  TreatAsAtomicUnit=on
  Constant : Constant  Value=-1
  Data Type Conversion : DataTypeConversion
  Switch : Switch  Criteria=u2 ~= 0  Threshold=1  ZeroCross=off
  WindowLogicOutput : Outport
  wires:
  OW/1 -> Data Type Conversion/1
  Switch/1 -> WindowLogicOutput/1
  WPos/1 -> Chart1/1(S)
  User/1 -> Chart1/2(UI)
  Constant/1 -> Switch/1
  Data Type Conversion/1 -> Switch/2
  Chart1/1(W) -> Switch/3

== system c00010M_harness/M048/Cyber/WL2 ==
  note: Sensors
  WPos : Inport
  User : Inport  Port=2
  OW : Inport  Port=3
  L : Inport  Port=4
  Chart1 : Stateflow chart  TreatAsAtomicUnit=on
  Constant : Constant  Value=-1
  Constant1 : Constant  Value=0
  Constant2 : Constant  Value=PosMinimaW3
  Data Type Conversion : DataTypeConversion
  Switch : Switch  Criteria=u2 ~= 0  Threshold=1  ZeroCross=off
  Switch1 : Switch  Criteria=u2 ~= 0
  WindowLogicOutput : Outport
  wires:
  Constant2/1 -> Chart1/3(PosMinW3)
  L/1 -> Switch1/2
  Data Type Conversion/1 -> Switch/2
  Constant/1 -> Switch/1
  Chart1/1(W) -> Switch1/3
  User/1 -> Chart1/2(UI)
  WPos/1 -> Chart1/1(S)
  Switch1/1 -> Switch/3
  Constant1/1 -> Switch1/1
  Switch/1 -> WindowLogicOutput/1
  OW/1 -> Data Type Conversion/1

== system c00010M_harness/M048/Physical/W ==
  WIn : Inport
  DC_Engine : Subsystem
  Discrete-Time Integrator : DiscreteIntegrator  InitialCondition=5  SampleTime=-1  LimitOutput=on  UpperSaturationLimit=5  LowerSaturationLimit=0  ICPrevOutput=DiscIntNeverNeededParam  ICPrevScaledInput=DiscIntNeverNeededParam
  WPos : Outport
  wires:
  WIn/1 -> DC_Engine/1(input)
  DC_Engine/1(Speed) -> Discrete-Time Integrator/1
  Discrete-Time Integrator/1 -> WPos/1

== system c00010M_harness/M048/Physical/W5 ==
  WIn : Inport
  DC_Engine : Subsystem
  Discrete-Time Integrator : DiscreteIntegrator  InitialCondition=5  SampleTime=-1  LimitOutput=on  UpperSaturationLimit=5  LowerSaturationLimit=0  ICPrevOutput=DiscIntNeverNeededParam  ICPrevScaledInput=DiscIntNeverNeededParam
  WPos : Outport
  wires:
  Discrete-Time Integrator/1 -> WPos/1
  DC_Engine/1(Speed) -> Discrete-Time Integrator/1
  WIn/1 -> DC_Engine/1(input)

== system c00010M_harness/M048/Physical/W6 ==
  WIn : Inport
  DC_Engine : Subsystem
  Discrete-Time Integrator : DiscreteIntegrator  InitialCondition=5  SampleTime=-1  LimitOutput=on  UpperSaturationLimit=5  LowerSaturationLimit=PosMinimaW3  ICPrevOutput=DiscIntNeverNeededParam  ICPrevScaledInput=DiscIntNeverNeededParam
  WPos : Outport
  wires:
  WIn/1 -> DC_Engine/1(input)
  DC_Engine/1(Speed) -> Discrete-Time Integrator/1
  Discrete-Time Integrator/1 -> WPos/1

== system c00010M_harness/M049/Cyber/Pri ==
  D : Inport
  P : Inport  Port=2
  Switch : Switch  Criteria=u2 ~= 0
  User : Outport
  wires:
  Switch/1 -> User/1
  D/1 -> Switch/2, Switch/1
  P/1 -> Switch/3

== system c00010M_harness/M049/Cyber/Pri1 ==
  D : Inport
  P : Inport  Port=2
  P1 : Inport  Port=3
  Switch : Switch  Criteria=u2 ~= 0
  Switch1 : Switch  Criteria=u2 ~= 0
  User : Outport
  wires:
  Switch1/1 -> Switch/3
  D/1 -> Switch/2, Switch/1
  P/1 -> Switch1/2, Switch1/1
  Switch/1 -> User/1
  P1/1 -> Switch1/3

== system c00010M_harness/M049/Cyber/WL ==
  note: Sensors
  WPos : Inport
  User : Inport  Port=2
  OW : Inport  Port=3
  Chart : Stateflow chart  TreatAsAtomicUnit=on
  Constant : Constant  Value=-1
  Data Type Conversion : DataTypeConversion
  Switch : Switch  Criteria=u2 ~= 0  Threshold=1  ZeroCross=off
  WindowLogicOutput : Outport
  wires:
  Data Type Conversion/1 -> Switch/2
  Constant/1 -> Switch/1
  User/1 -> Chart/2(UI)
  WPos/1 -> Chart/1(S)
  Switch/1 -> WindowLogicOutput/1
  OW/1 -> Data Type Conversion/1
  Chart/1(W) -> Switch/3

== system c00010M_harness/M049/Cyber/WL1 ==
  note: Sensors
  WPos : Inport
  User : Inport  Port=2
  OW : Inport  Port=3
  Chart1 : Stateflow chart  TreatAsAtomicUnit=on
  Constant : Constant  Value=-1
  Data Type Conversion : DataTypeConversion
  Switch : Switch  Criteria=u2 ~= 0  Threshold=1  ZeroCross=off
  WindowLogicOutput : Outport
  wires:
  OW/1 -> Data Type Conversion/1
  Switch/1 -> WindowLogicOutput/1
  WPos/1 -> Chart1/1(S)
  User/1 -> Chart1/2(UI)
  Constant/1 -> Switch/1
  Data Type Conversion/1 -> Switch/2
  Chart1/1(W) -> Switch/3

== system c00010M_harness/M049/Cyber/WL2 ==
  note: Sensors
  WPos : Inport
  User : Inport  Port=2
  OW : Inport  Port=3
  L : Inport  Port=4
  Chart1 : Stateflow chart  TreatAsAtomicUnit=on
  Constant : Constant  Value=-1
  Constant1 : Constant  Value=0
  Constant2 : Constant  Value=PosMinimaW3
  Data Type Conversion : DataTypeConversion
  Switch : Switch  Criteria=u2 ~= 0  Threshold=1  ZeroCross=off
  Switch1 : Switch  Criteria=u2 ~= 0
  WindowLogicOutput : Outport
  wires:
  Constant2/1 -> Chart1/3(PosMinW3)
  L/1 -> Switch1/2
  Data Type Conversion/1 -> Switch/2
  Constant/1 -> Switch/1
  Chart1/1(W) -> Switch1/3
  User/1 -> Chart1/2(UI)
  WPos/1 -> Chart1/1(S)
  Switch1/1 -> Switch/3
  Constant1/1 -> Switch1/1
  Switch/1 -> WindowLogicOutput/1
  OW/1 -> Data Type Conversion/1

== system c00010M_harness/M049/Physical/W ==
  WIn : Inport
  DC_Engine : Subsystem
  Discrete-Time Integrator : DiscreteIntegrator  InitialCondition=5  SampleTime=-1  LimitOutput=on  UpperSaturationLimit=5  LowerSaturationLimit=0  ICPrevOutput=DiscIntNeverNeededParam  ICPrevScaledInput=DiscIntNeverNeededParam
  WPos : Outport
  wires:
  WIn/1 -> DC_Engine/1(input)
  DC_Engine/1(Speed) -> Discrete-Time Integrator/1
  Discrete-Time Integrator/1 -> WPos/1

== system c00010M_harness/M049/Physical/W5 ==
  WIn : Inport
  DC_Engine : Subsystem
  Discrete-Time Integrator : DiscreteIntegrator  InitialCondition=5  SampleTime=-1  LimitOutput=on  UpperSaturationLimit=5  LowerSaturationLimit=0  ICPrevOutput=DiscIntNeverNeededParam  ICPrevScaledInput=DiscIntNeverNeededParam
  WPos : Outport
  wires:
  Discrete-Time Integrator/1 -> WPos/1
  DC_Engine/1(Speed) -> Discrete-Time Integrator/1
  WIn/1 -> DC_Engine/1(input)

== system c00010M_harness/M049/Physical/W6 ==
  WIn : Inport
  DC_Engine : Subsystem
  Discrete-Time Integrator : DiscreteIntegrator  InitialCondition=5  SampleTime=-1  LimitOutput=on  UpperSaturationLimit=5  LowerSaturationLimit=PosMinimaW3  ICPrevOutput=DiscIntNeverNeededParam  ICPrevScaledInput=DiscIntNeverNeededParam
  WPos : Outport
  wires:
  WIn/1 -> DC_Engine/1(input)
  DC_Engine/1(Speed) -> Discrete-Time Integrator/1
  Discrete-Time Integrator/1 -> WPos/1

== system c00010M_harness/M051/Cyber/Pri ==
  D : Inport
  P : Inport  Port=2
  Switch : Switch  Criteria=u2 ~= 0
  User : Outport
  wires:
  Switch/1 -> User/1
  D/1 -> Switch/2, Switch/1
  P/1 -> Switch/3

== system c00010M_harness/M051/Cyber/Pri1 ==
  D : Inport
  P : Inport  Port=2
  P1 : Inport  Port=3
  Switch : Switch  Criteria=u2 ~= 0
  Switch1 : Switch  Criteria=u2 ~= 0
  User : Outport
  wires:
  Switch1/1 -> Switch/3
  D/1 -> Switch/2, Switch/1
  P/1 -> Switch1/2, Switch1/1
  Switch/1 -> User/1
  P1/1 -> Switch1/3

== system c00010M_harness/M051/Cyber/WL ==
  note: Sensors
  WPos : Inport
  User : Inport  Port=2
  OW : Inport  Port=3
  Chart : Stateflow chart  TreatAsAtomicUnit=on
  Constant : Constant  Value=-1
  Data Type Conversion : DataTypeConversion
  Switch : Switch  Criteria=u2 ~= 0  Threshold=1  ZeroCross=off
  WindowLogicOutput : Outport
  wires:
  Data Type Conversion/1 -> Switch/2
  Constant/1 -> Switch/1
  User/1 -> Chart/2(UI)
  WPos/1 -> Chart/1(S)
  Switch/1 -> WindowLogicOutput/1
  OW/1 -> Data Type Conversion/1
  Chart/1(W) -> Switch/3

== system c00010M_harness/M051/Cyber/WL1 ==
  note: Sensors
  WPos : Inport
  User : Inport  Port=2
  OW : Inport  Port=3
  Chart1 : Stateflow chart  TreatAsAtomicUnit=on
  Constant : Constant  Value=-1
  Data Type Conversion : DataTypeConversion
  Switch : Switch  Criteria=u2 ~= 0  Threshold=1  ZeroCross=off
  WindowLogicOutput : Outport
  wires:
  OW/1 -> Data Type Conversion/1
  Switch/1 -> WindowLogicOutput/1
  WPos/1 -> Chart1/1(S)
  User/1 -> Chart1/2(UI)
  Constant/1 -> Switch/1
  Data Type Conversion/1 -> Switch/2
  Chart1/1(W) -> Switch/3

== system c00010M_harness/M051/Cyber/WL2 ==
  note: Sensors
  WPos : Inport
  User : Inport  Port=2
  OW : Inport  Port=3
  L : Inport  Port=4
  Chart1 : Stateflow chart  TreatAsAtomicUnit=on
  Constant : Constant  Value=-1
  Constant1 : Constant  Value=0
  Constant2 : Constant  Value=PosMinimaW3
  Data Type Conversion : DataTypeConversion
  Switch : Switch  Criteria=u2 ~= 0  Threshold=1  ZeroCross=off
  Switch1 : Switch  Criteria=u2 ~= 0
  WindowLogicOutput : Outport
  wires:
  Constant2/1 -> Chart1/3(PosMinW3)
  L/1 -> Switch1/2
  Data Type Conversion/1 -> Switch/2
  Constant/1 -> Switch/1
  Chart1/1(W) -> Switch1/3
  User/1 -> Chart1/2(UI)
  WPos/1 -> Chart1/1(S)
  Switch1/1 -> Switch/3
  Constant1/1 -> Switch1/1
  Switch/1 -> WindowLogicOutput/1
  OW/1 -> Data Type Conversion/1

== system c00010M_harness/M051/Physical/W ==
  WIn : Inport
  DC_Engine : Subsystem
  Discrete-Time Integrator : DiscreteIntegrator  InitialCondition=5  SampleTime=-1  LimitOutput=on  UpperSaturationLimit=5  LowerSaturationLimit=0  ICPrevOutput=DiscIntNeverNeededParam  ICPrevScaledInput=DiscIntNeverNeededParam
  WPos : Outport
  wires:
  WIn/1 -> DC_Engine/1(input)
  DC_Engine/1(Speed) -> Discrete-Time Integrator/1
  Discrete-Time Integrator/1 -> WPos/1

== system c00010M_harness/M051/Physical/W5 ==
  WIn : Inport
  DC_Engine : Subsystem
  Discrete-Time Integrator : DiscreteIntegrator  InitialCondition=5  SampleTime=-1  LimitOutput=on  UpperSaturationLimit=5  LowerSaturationLimit=0  ICPrevOutput=DiscIntNeverNeededParam  ICPrevScaledInput=DiscIntNeverNeededParam
  WPos : Outport
  wires:
  Discrete-Time Integrator/1 -> WPos/1
  DC_Engine/1(Speed) -> Discrete-Time Integrator/1
  WIn/1 -> DC_Engine/1(input)

== system c00010M_harness/M051/Physical/W6 ==
  WIn : Inport
  DC_Engine : Subsystem
  Discrete-Time Integrator : DiscreteIntegrator  InitialCondition=5  SampleTime=-1  LimitOutput=on  UpperSaturationLimit=5  LowerSaturationLimit=PosMinimaW3  ICPrevOutput=DiscIntNeverNeededParam  ICPrevScaledInput=DiscIntNeverNeededParam
  WPos : Outport
  wires:
  WIn/1 -> DC_Engine/1(input)
  DC_Engine/1(Speed) -> Discrete-Time Integrator/1
  Discrete-Time Integrator/1 -> WPos/1

== system c00010M_harness/M052/Cyber/Pri ==
  D : Inport
  P : Inport  Port=2
  Switch : Switch  Criteria=u2 ~= 0
  User : Outport
  wires:
  Switch/1 -> User/1
  D/1 -> Switch/2, Switch/1
  P/1 -> Switch/3

== system c00010M_harness/M052/Cyber/Pri1 ==
  D : Inport
  P : Inport  Port=2
  P1 : Inport  Port=3
  Switch : Switch  Criteria=u2 ~= 0
  Switch1 : Switch  Criteria=u2 ~= 0
  User : Outport
  wires:
  Switch1/1 -> Switch/3
  D/1 -> Switch/2, Switch/1
  P/1 -> Switch1/2, Switch1/1
  Switch/1 -> User/1
  P1/1 -> Switch1/3

== system c00010M_harness/M052/Cyber/WL ==
  note: Sensors
  WPos : Inport
  User : Inport  Port=2
  OW : Inport  Port=3
  Chart : Stateflow chart  TreatAsAtomicUnit=on
  Constant : Constant  Value=-1
  Data Type Conversion : DataTypeConversion
  Switch : Switch  Criteria=u2 ~= 0  Threshold=1  ZeroCross=off
  WindowLogicOutput : Outport
  wires:
  Data Type Conversion/1 -> Switch/2
  Constant/1 -> Switch/1
  User/1 -> Chart/2(UI)
  WPos/1 -> Chart/1(S)
  Switch/1 -> WindowLogicOutput/1
  OW/1 -> Data Type Conversion/1
  Chart/1(W) -> Switch/3

== system c00010M_harness/M052/Cyber/WL1 ==
  note: Sensors
  WPos : Inport
  User : Inport  Port=2
  OW : Inport  Port=3
  Chart1 : Stateflow chart  TreatAsAtomicUnit=on
  Constant : Constant  Value=-1
  Data Type Conversion : DataTypeConversion
  Switch : Switch  Criteria=u2 ~= 0  Threshold=1  ZeroCross=off
  WindowLogicOutput : Outport
  wires:
  OW/1 -> Data Type Conversion/1
  Switch/1 -> WindowLogicOutput/1
  WPos/1 -> Chart1/1(S)
  User/1 -> Chart1/2(UI)
  Constant/1 -> Switch/1
  Data Type Conversion/1 -> Switch/2
  Chart1/1(W) -> Switch/3

== system c00010M_harness/M052/Cyber/WL2 ==
  note: Sensors
  WPos : Inport
  User : Inport  Port=2
  OW : Inport  Port=3
  L : Inport  Port=4
  Chart1 : Stateflow chart  TreatAsAtomicUnit=on
  Constant : Constant  Value=-1
  Constant1 : Constant  Value=0
  Constant2 : Constant  Value=PosMinimaW3
  Data Type Conversion : DataTypeConversion
  Switch : Switch  Criteria=u2 ~= 0  Threshold=1  ZeroCross=off
  Switch1 : Switch  Criteria=u2 ~= 0
  WindowLogicOutput : Outport
  wires:
  Constant2/1 -> Chart1/3(PosMinW3)
  L/1 -> Switch1/2
  Data Type Conversion/1 -> Switch/2
  Constant/1 -> Switch/1
  Chart1/1(W) -> Switch1/3
  User/1 -> Chart1/2(UI)
  WPos/1 -> Chart1/1(S)
  Switch1/1 -> Switch/3
  Constant1/1 -> Switch1/1
  Switch/1 -> WindowLogicOutput/1
  OW/1 -> Data Type Conversion/1

== system c00010M_harness/M052/Physical/W ==
  WIn : Inport
  DC_Engine : Subsystem
  Discrete-Time Integrator : DiscreteIntegrator  InitialCondition=5  SampleTime=-1  LimitOutput=on  UpperSaturationLimit=5  LowerSaturationLimit=0  ICPrevOutput=DiscIntNeverNeededParam  ICPrevScaledInput=DiscIntNeverNeededParam
  WPos : Outport
  wires:
  WIn/1 -> DC_Engine/1(input)
  DC_Engine/1(Speed) -> Discrete-Time Integrator/1
  Discrete-Time Integrator/1 -> WPos/1

== system c00010M_harness/M052/Physical/W5 ==
  WIn : Inport
  DC_Engine : Subsystem
  Discrete-Time Integrator : DiscreteIntegrator  InitialCondition=5  SampleTime=-1  LimitOutput=on  UpperSaturationLimit=5  LowerSaturationLimit=0  ICPrevOutput=DiscIntNeverNeededParam  ICPrevScaledInput=DiscIntNeverNeededParam
  WPos : Outport
  wires:
  Discrete-Time Integrator/1 -> WPos/1
  DC_Engine/1(Speed) -> Discrete-Time Integrator/1
  WIn/1 -> DC_Engine/1(input)

== system c00010M_harness/M052/Physical/W6 ==
  WIn : Inport
  DC_Engine : Subsystem
  Discrete-Time Integrator : DiscreteIntegrator  InitialCondition=5  SampleTime=-1  LimitOutput=on  UpperSaturationLimit=5  LowerSaturationLimit=PosMinimaW3  ICPrevOutput=DiscIntNeverNeededParam  ICPrevScaledInput=DiscIntNeverNeededParam
  WPos : Outport
  wires:
  WIn/1 -> DC_Engine/1(input)
  DC_Engine/1(Speed) -> Discrete-Time Integrator/1
  Discrete-Time Integrator/1 -> WPos/1

== system c00010M_harness/M053/Cyber/Pri ==
  D : Inport
  P : Inport  Port=2
  Switch : Switch  Criteria=u2 ~= 0
  User : Outport
  wires:
  Switch/1 -> User/1
  D/1 -> Switch/2, Switch/1
  P/1 -> Switch/3

== system c00010M_harness/M053/Cyber/Pri1 ==
  D : Inport
  P : Inport  Port=2
  P1 : Inport  Port=3
  Switch : Switch  Criteria=u2 ~= 0
  Switch1 : Switch  Criteria=u2 ~= 0
  User : Outport
  wires:
  Switch1/1 -> Switch/3
  D/1 -> Switch/2, Switch/1
  P/1 -> Switch1/2, Switch1/1
  Switch/1 -> User/1
  P1/1 -> Switch1/3

== system c00010M_harness/M053/Cyber/WL ==
  note: Sensors
  WPos : Inport
  User : Inport  Port=2
  OW : Inport  Port=3
  Chart : Stateflow chart  TreatAsAtomicUnit=on
  Constant : Constant  Value=-1
  Data Type Conversion : DataTypeConversion
  Switch : Switch  Criteria=u2 ~= 0  Threshold=1  ZeroCross=off
  WindowLogicOutput : Outport
  wires:
  Data Type Conversion/1 -> Switch/2
  Constant/1 -> Switch/1
  User/1 -> Chart/2(UI)
  WPos/1 -> Chart/1(S)
  Switch/1 -> WindowLogicOutput/1
  OW/1 -> Data Type Conversion/1
  Chart/1(W) -> Switch/3

== system c00010M_harness/M053/Cyber/WL1 ==
  note: Sensors
  WPos : Inport
  User : Inport  Port=2
  OW : Inport  Port=3
  Chart1 : Stateflow chart  TreatAsAtomicUnit=on
  Constant : Constant  Value=-1
  Data Type Conversion : DataTypeConversion
  Switch : Switch  Criteria=u2 ~= 0  Threshold=1  ZeroCross=off
  WindowLogicOutput : Outport
  wires:
  OW/1 -> Data Type Conversion/1
  Switch/1 -> WindowLogicOutput/1
  WPos/1 -> Chart1/1(S)
  User/1 -> Chart1/2(UI)
  Constant/1 -> Switch/1
  Data Type Conversion/1 -> Switch/2
  Chart1/1(W) -> Switch/3

== system c00010M_harness/M053/Cyber/WL2 ==
  note: Sensors
  WPos : Inport
  User : Inport  Port=2
  OW : Inport  Port=3
  L : Inport  Port=4
  Chart1 : Stateflow chart  TreatAsAtomicUnit=on
  Constant : Constant  Value=-1
  Constant1 : Constant  Value=0
  Constant2 : Constant  Value=PosMinimaW3
  Data Type Conversion : DataTypeConversion
  Switch : Switch  Criteria=u2 ~= 0  Threshold=1  ZeroCross=off
  Switch1 : Switch  Criteria=u2 ~= 0
  WindowLogicOutput : Outport
  wires:
  Constant2/1 -> Chart1/3(PosMinW3)
  L/1 -> Switch1/2
  Data Type Conversion/1 -> Switch/2
  Constant/1 -> Switch/1
  Chart1/1(W) -> Switch1/3
  User/1 -> Chart1/2(UI)
  WPos/1 -> Chart1/1(S)
  Switch1/1 -> Switch/3
  Constant1/1 -> Switch1/1
  Switch/1 -> WindowLogicOutput/1
  OW/1 -> Data Type Conversion/1
